simulink model "sysp3"  (R2023a)
settings: Solver=ode15s  StartTime=0.0  StopTime=30  MaxStep=1E-3  RelTol=1e-3
libraries: slpidlib x1
settings Model: Creator=Ariel  LastModifiedBy=cesar
settings SolverCC: MaxConsecutiveZCs=10
settings DataIOCC: ReturnWorkspaceOutputs=off  TimeSaveName=t
settings DebuggingCC: AlgebraicLoopMsg=none  ArtificialAlgebraicLoopMsg=none  MaxConsecutiveZCsMsg=none  ModelReferenceExtraNoncontSigs=none  OperatingPointInterfaceChecksumMismatchMsg=none

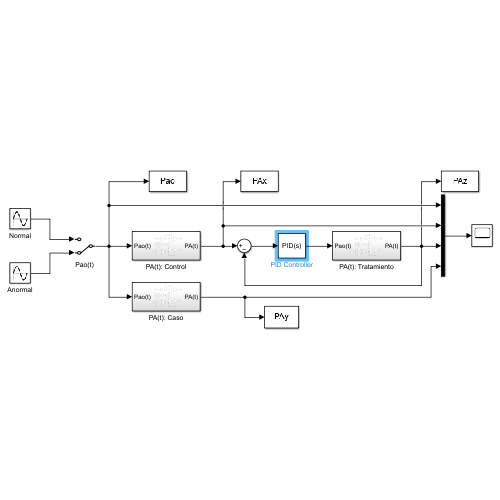
[thumbnail: Simulink's stored preview of the top-level diagram]
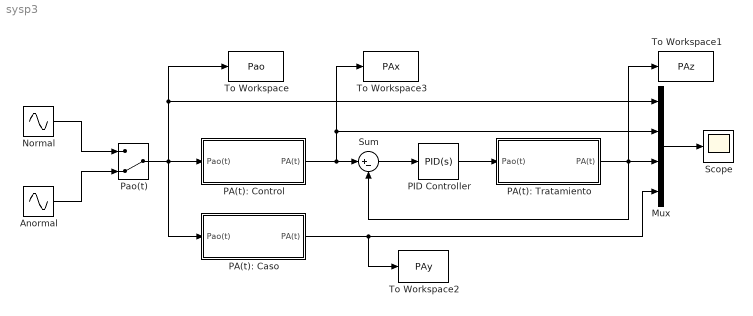
== system sysp3 ==
  Anormal : Sin  Amplitude=1.5  Frequency=pi  SampleTime=0
  Mux : Mux
  Normal : Sin  Amplitude=2.5  Frequency=pi/2  SampleTime=0
  PA(t): Caso : Subsystem
  PA(t): Control : Subsystem
  PA(t): Tratamiento : Subsystem
  PID Controller : slpidlib/PID Controller  Controller=PID  Form=Parallel  TimeDomain=Continuous-time  UseExternalTs=off  SampleTime=-1  IntegratorMethod=Forward Euler  FilterMethod=Forward Euler  ControllerParametersSource=internal  P=171.2458  I=4040.7036  UseKiTs=off  D=0.9276  N=14035.6841  UseFilter=on  TunerSelectOption=Transfer Function Based (PID Tuner App)  InitialConditionSource=internal  InitialConditionForIntegrator=0  InitialConditionForFilter=0  DifferentiatorICPrevScaledInput=0  ExternalReset=none  TrackingMode=off  Kt=1  LimitOutput=off  SatLimitsSource=internal  UpperSaturationLimit=inf  LowerSaturationLimit=-inf  LinearizeAsGain=on  AntiWindupMode=none  Kb=1  LimitIntegrator=off  UpperIntegratorSaturationLimit=inf  LowerIntegratorSaturationLimit=-inf  POutMin=[]  POutMax=[]  IOutMin=[]  IOutMax=[]  DOutMin=[]  DOutMax=[]  NOutMin=[]  NOutMax=[]  SumOutMin=[]  SumOutMax=[]  SaturationOutMin=[]  SaturationOutMax=[]  PParamMin=[]  PParamMax=[]  IParamMin=[]  IParamMax=[]  DParamMin=[]  DParamMax=[]  NParamMin=[]  NParamMax=[]  KbParamMin=[]  KbParamMax=[]  KtParamMin=[]  KtParamMax=[]  KbOutMin=[]  KbOutMax=[]  KtOutMin=[]  KtOutMax=[]  IntegratorOutMin=[]  IntegratorOutMax=[]  FilterOutMin=[]  FilterOutMax=[]  SumI1OutMin=[]  SumI1OutMax=[]  SumI2OutMin=[]  SumI2OutMax=[]  SumI3OutMin=[]  SumI3OutMax=[]  SumI4OutMin=[]  SumI4OutMax=[]  SumDOutMin=[]  SumDOutMax=[]  DifferentiatorOutMin=[]  DifferentiatorOutMax=[]  FilterDiffOutCoefMin=[]  FilterDiffOutCoefMax=[]  ReciprocalOutMin=[]  ReciprocalOutMax=[]  SumDenOutMin=[]  SumDenOutMax=[]  SumNumOutMin=[]  SumNumOutMax=[]  DivideOutMin=[]  DivideOutMax=[]  UdiffTsProdOutMin=[]  UdiffTsProdOutMax=[]  NTsProdOutMin=[]  NTsProdOutMax=[]  UintegralTsProdOutMin=[]  UintegralTsProdOutMax=[]  UngainTsProdOutMin=[]  UngainTsProdOutMax=[]  ClampingZeroOutDataTypeStr=Inherit: Inherit via back propagation  ClampingZeroOutMin=[]  ClampingZeroOutMax=[]  FilterDenConstantOutDataTypeStr=Inherit: Inherit via back propagation  FilterDenConstantOutMin=[]  FilterDenConstantOutMax=[]  PCopyOutDataTypeStr=Inherit: Inherit via back propagation  PCopyOutMin=[]  PCopyOutMax=[]  NCopyOutDataTypeStr=Inherit: Inherit via back propagation  NCopyOutMin=[]  NCopyOutMax=[]  IntegratorContinuousStateAttributes=''  IntegratorStateMustResolveToSignalObject=off  IntegratorRTWStateStorageClass=Auto  FilterContinuousStateAttributes=''  FilterStateMustResolveToSignalObject=off  FilterRTWStateStorageClass=Auto  ParallelPVariant=InternalParameters  IdealPVariant=Disabled  IVariant=InternalParameters  DVariant=InternalParameters  IntegratorVariant=Continuous  SatVariant=Disabled  AWVariant=Passthrough  PCopyVariant=Disabled  TRVariant=Disabled  FdbkBlocksVariant=Forward  IdealPFdbkVariant=Disabled  SatFdbkVariant=Disabled  DerivativeFilterVariant=ContFilter  NVariant=InternalParameters  NCopyVariant=Disabled  FilterICVariant=InternalICsFilter  IntegratorICVariant=InternalICs  ExternalResetVariant=Disabled  TRSumVariant=Passthrough  SumFdbkVariant=Disabled  SumVariant=Sum_PID  TsampFilterVariant=InternalTs  TsampNgainVariant=Passthrough  TsampIntegralVariant=Disabled_SignalSpec  ExternalSaturationOutDataTypeStr=Inherit: Same as second input
  Pao(t) : ManualSwitch  CurrentSetting=0
  Scope : Scope
  Sum : Sum  Inputs=|+-
  To Workspace : ToWorkspace  VariableName=Pao  SaveFormat=Timeseries  SampleTime=-1
  To Workspace1 : ToWorkspace  VariableName=PAz  SaveFormat=Timeseries  SampleTime=-1
  To Workspace2 : ToWorkspace  VariableName=PAy  SaveFormat=Timeseries  SampleTime=-1
  To Workspace3 : ToWorkspace  VariableName=PAx  SaveFormat=Timeseries  SampleTime=-1
  wires:
  Mux/1 -> Scope/1
  Pao(t)/1 -> PA(t): Caso/1(Pao(t)), PA(t): Control/1(Pao(t)), Mux/1, To Workspace/1
  Normal/1 -> Pao(t)/1
  Anormal/1 -> Pao(t)/2
  Sum/1 -> PID Controller/1
  PA(t): Control/1(PA(t)) -> Mux/2, To Workspace3/1, Sum/1
  PID Controller/1 -> PA(t): Tratamiento/1(Pao(t))
  PA(t): Caso/1(PA(t)) -> Mux/4, To Workspace2/1
  PA(t): Tratamiento/1(PA(t)) -> Mux/3, To Workspace1/1, Sum/2

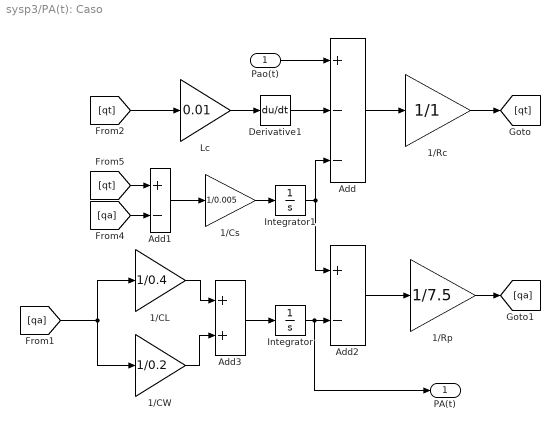
== system sysp3/PA(t): Caso ==
  Pao(t) : Inport
  1/CL : Gain  Gain=1/0.4
  1/CW : Gain  Gain=1/0.2
  1/Cs : Gain  Gain=1/0.005
  1/Rc : Gain  Gain=1/1
  1/Rp : Gain  Gain=1/7.5
  Add : Sum  Inputs=+--
  Add1 : Sum  Inputs=+-
  Add2 : Sum  Inputs=+-
  Add3 : Sum
  Derivative1 : Derivative
  Integrator : Integrator
  Integrator1 : Integrator
  Lc : Gain  Gain=0.01
  PA(t) : Outport
  wires:
  Pao(t)/1 -> Add/1
  1/CL/1 -> Add3/1
  Add2/1 -> 1/Rp/1
  1/CW/1 -> Add3/2
  1/Rp/1 -> [qa]
  [qa] -> Add1/2
  [qt] -> Add1/1
  1/Rc/1 -> [qt]
  Add/1 -> 1/Rc/1
  [qa] -> 1/CW/1, 1/CL/1
  Add3/1 -> Integrator/1
  Integrator/1 -> PA(t)/1, Add2/2
  Lc/1 -> Derivative1/1
  Derivative1/1 -> Add/2
  [qt] -> Lc/1
  Add1/1 -> 1/Cs/1
  1/Cs/1 -> Integrator1/1
  Integrator1/1 -> Add2/1, Add/3

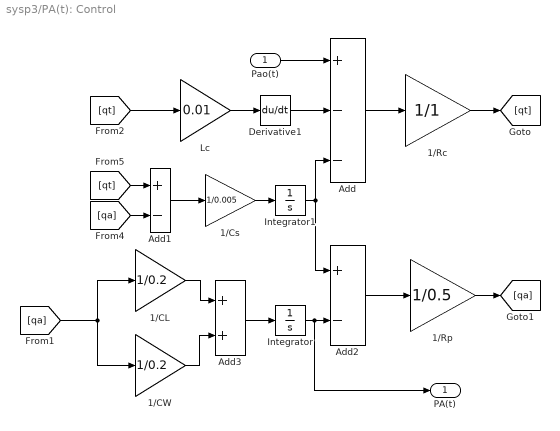
== system sysp3/PA(t): Control ==
  Pao(t) : Inport
  1/CL : Gain  Gain=1/0.2
  1/CW : Gain  Gain=1/0.2
  1/Cs : Gain  Gain=1/0.005
  1/Rc : Gain  Gain=1/1
  1/Rp : Gain  Gain=1/0.5
  Add : Sum  Inputs=+--
  Add1 : Sum  Inputs=+-
  Add2 : Sum  Inputs=+-
  Add3 : Sum
  Derivative1 : Derivative
  Integrator : Integrator
  Integrator1 : Integrator
  Lc : Gain  Gain=0.01
  PA(t) : Outport
  wires:
  Pao(t)/1 -> Add/1
  1/CL/1 -> Add3/1
  Add2/1 -> 1/Rp/1
  1/CW/1 -> Add3/2
  1/Rp/1 -> [qa]
  [qa] -> Add1/2
  [qt] -> Add1/1
  1/Rc/1 -> [qt]
  Add/1 -> 1/Rc/1
  [qa] -> 1/CW/1, 1/CL/1
  Add3/1 -> Integrator/1
  Integrator/1 -> PA(t)/1, Add2/2
  Lc/1 -> Derivative1/1
  Derivative1/1 -> Add/2
  [qt] -> Lc/1
  Add1/1 -> 1/Cs/1
  1/Cs/1 -> Integrator1/1
  Integrator1/1 -> Add2/1, Add/3

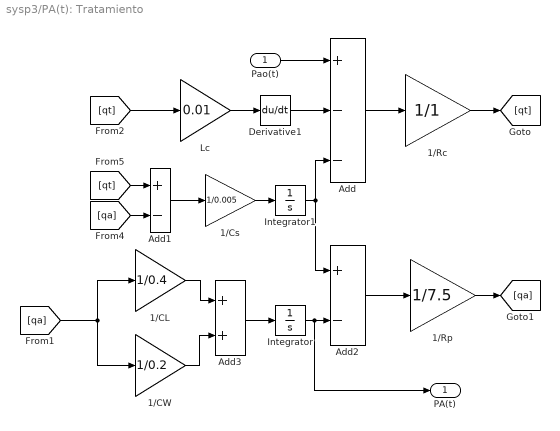
== system sysp3/PA(t): Tratamiento ==
  Pao(t) : Inport
  1/CL : Gain  Gain=1/0.4
  1/CW : Gain  Gain=1/0.2
  1/Cs : Gain  Gain=1/0.005
  1/Rc : Gain  Gain=1/1
  1/Rp : Gain  Gain=1/7.5
  Add : Sum  Inputs=+--
  Add1 : Sum  Inputs=+-
  Add2 : Sum  Inputs=+-
  Add3 : Sum
  Derivative1 : Derivative
  Integrator : Integrator
  Integrator1 : Integrator
  Lc : Gain  Gain=0.01
  PA(t) : Outport
  wires:
  Pao(t)/1 -> Add/1
  1/CL/1 -> Add3/1
  Add2/1 -> 1/Rp/1
  1/CW/1 -> Add3/2
  1/Rp/1 -> [qa]
  [qa] -> Add1/2
  [qt] -> Add1/1
  1/Rc/1 -> [qt]
  Add/1 -> 1/Rc/1
  [qa] -> 1/CW/1, 1/CL/1
  Add3/1 -> Integrator/1
  Integrator/1 -> PA(t)/1, Add2/2
  Lc/1 -> Derivative1/1
  Derivative1/1 -> Add/2
  [qt] -> Lc/1
  Add1/1 -> 1/Cs/1
  1/Cs/1 -> Integrator1/1
  Integrator1/1 -> Add2/1, Add/3
